simulink model "master_slave_example"  (R2020b)
settings: Solver=ode45  StartTime=0.0  StopTime=2  MaxStep=1e-4  RelTol=1e-3
libraries: simulink x2
settings Model: Creator=carma  LastModifiedBy=Acer
settings DataIOCC: ReturnWorkspaceOutputs=off
settings DebuggingCC: ArithmeticOperatorsInVariantConditions=warning
settings SFSimCC: SimUseLocalCustomCode=off  CustomCodeUndefinedFunction=UseInterfaceOnly
settings RTWCC: RTWUseLocalCustomCode=off

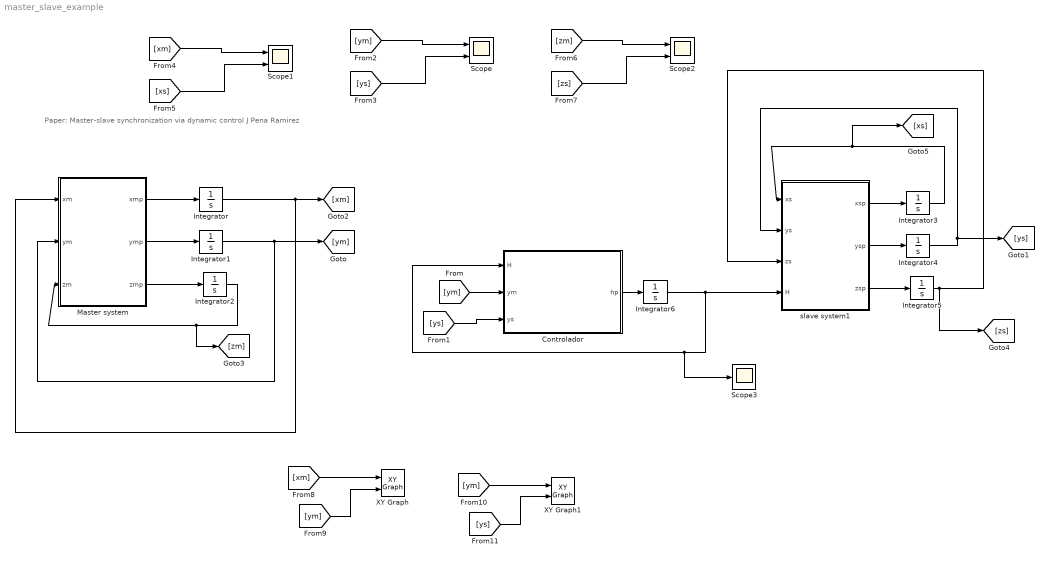
== system master_slave_example ==
  note: Paper: Master-slave synchronization via dynamic control J Pena Ramirez
  Controlador : MATLAB Function  TreatAsAtomicUnit=on
  Integrator{,1..6} (7 alike) : Integrator
  Master system : MATLAB Function  TreatAsAtomicUnit=on
  Scope : Scope  NumInputPorts=2
  Scope1 : Scope  NumInputPorts=2
  Scope2 : Scope  NumInputPorts=2
  Scope3 : Scope
  XY Graph : simulink/Sinks/XY Graph  xmin=-5  xmax=6  ymin=-6  ymax=4  st=-1
  XY Graph1 : simulink/Sinks/XY Graph  xmin=-8  xmax=6  ymin=-8  ymax=6  st=-1
  slave system1 : MATLAB Function  TreatAsAtomicUnit=on
  wires:
  Master system/1(xmp) -> Integrator/1
  Master system/2(ymp) -> Integrator1/1
  Master system/3(zmp) -> Integrator2/1
  Integrator2/1 -> [zm], Master system/3(zm)
  Integrator1/1 -> [ym], Master system/2(ym)
  slave system1/2(ysp) -> Integrator4/1
  slave system1/3(zsp) -> Integrator5/1
  slave system1/1(xsp) -> Integrator3/1
  Integrator3/1 -> [xs], slave system1/1(xs)
  Integrator4/1 -> [ys], slave system1/2(ys)
  Integrator5/1 -> [zs], slave system1/3(zs)
  [ym] -> Controlador/2(ym)
  [ys] -> Controlador/3(ys)
  Controlador/1(hp) -> Integrator6/1
  Integrator6/1 -> Scope3/1, Controlador/1(H), slave system1/4(H)
  [ym] -> Scope/1
  [ys] -> Scope/2
  [xs] -> Scope1/2
  [xm] -> Scope1/1
  [zs] -> Scope2/2
  [zm] -> Scope2/1
  Integrator/1 -> [xm], Master system/1(xm)
  [xm] -> XY Graph/1
  [ym] -> XY Graph/2
  [ym] -> XY Graph1/1
  [ys] -> XY Graph1/2

== matlab function master_slave_example/slave system1 ==
  data: xs input; ys input; zs input; H input; xsp output; ysp output; zsp output
function [xsp,ysp,zsp] = fcn(xs,ys,zs,H)

% a=0.2;
% b=0.2;
% c=5.7;
a=0.2;
b=0.2;
c=5.7;
wc=100e3*22e-9;

xsp=(-ys-zs-H)/wc;
ysp=(xs+a*ys)/wc;
zsp=(b/2+zs*(2*xs-c))/wc;

% xsp=(-ys/2-zs/2-H/2)/wc;
% ysp=(xs/2+a*ys/2)/wc;
% zsp=(b/2+zs/2*(2*xs/2-c))/wc;

== matlab function master_slave_example/Master system ==
  data: xm input; xmp output; ym input; zm input; ymp output; zmp output
function [xmp,ymp,zmp] = fcn(xm,ym,zm)

a=0.2;
b=0.2;
c=5.7;
wc=100e3*22e-9;

xmp=(-ym-zm)/wc;
ymp=(xm+a*ym)/wc;
zmp=(b/2+zm*(2*xm-c))/wc;

% xmp=(-ym/2-zm/2)/wc;
% ymp=(xm/2+a*ym/2)/wc;
% zmp=(b/2+zm/2*(2*xm/2-c))/wc;

== matlab function master_slave_example/Controlador ==
  data: H input; hp output; ym input; ys input
function hp = fcn(H,ym,ys)

wc=100e3*22e-9;
alpha=1;
k=-0.7;

% alpha=3;
%k=0;
% k=-0.9;
hp=(-alpha*H-k*(ym-ys))/wc;
% hp=(-alpha*H/2-k*(ym/2-ys/2))/wc;
